simulink model "main"  (R2016b)
settings: Solver=VariableStepAuto  StartTime=0.0  StopTime=0.4  FixedStep=2e-4  RelTol=1e-3
values from neighbouring files (symbols this model uses):
  TsN = 1e-5    (= 1e-05)    [initiateSimulation.m]
undefined symbols (not defined in the file or in its folder): denGc, denGp, numGc, numGp
libraries: simulink x1, model_controller x1
settings Model: Creator=Dai Luyao  LastModifiedBy=Dai Luyao

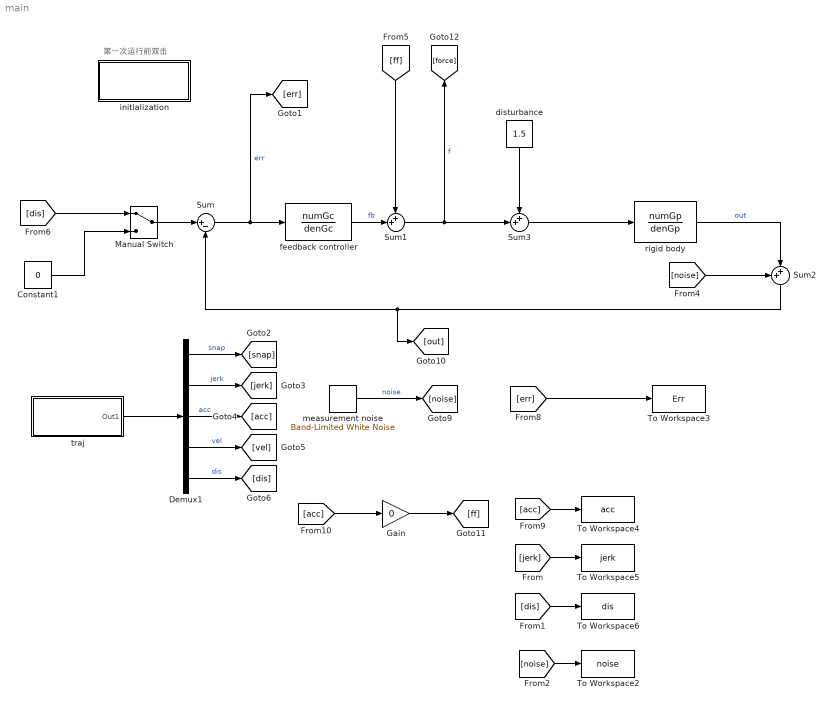
== system main ==
  note: 第一次运行前双击
  Constant1 : Constant  Value=0
  Demux1 : Demux  Outputs=5
  Gain : Gain  Gain=0
  Manual Switch : ManualSwitch
  Sum : Sum  Inputs=|+-
  Sum1 : Sum  Inputs=++|
  Sum2 : Sum  Inputs=++|
  Sum3 : Sum  Inputs=++|
  To Workspace2 : ToWorkspace  VariableName=noise  SaveFormat=Structure With Time  SampleTime=-1
  To Workspace3 : ToWorkspace  VariableName=Err  SaveFormat=Structure With Time  SampleTime=-1
  To Workspace4 : ToWorkspace  VariableName=acc  SaveFormat=Structure With Time  SampleTime=-1
  To Workspace5 : ToWorkspace  VariableName=jerk  SaveFormat=Structure With Time  SampleTime=-1
  To Workspace6 : ToWorkspace  VariableName=dis  SaveFormat=Structure With Time  SampleTime=-1
  disturbance : Constant  Value=1.5
  feedback controller : TransferFcn  Numerator=numGc  Denominator=denGc
  initialization : Subsystem
      settings: OpenFcn=initiateSimulation;  MoveFcn=edit initiateSimulation;
  measurement noise : simulink/Sources/Band-Limited White Noise  Cov=noisePower  Ts=TsN  seed=[23341]
  rigid body : TransferFcn  Numerator=numGp  Denominator=denGp
  traj : Subsystem  BlockChoice=zero
      link override 3rd order traj: j=800  v=0.25  x=0.06  a=10
      link override 4th order traj: a=10  v=0.25
      settings: AttributesFormatString=%<BlockChoice>  TemplateBlock=model_controller/Profile Generators/traj  MemberBlocks=2nd order traj,3rd order traj,4th order traj,step,zero
  wires:
  Sum/1 -> feedback controller/1, [err]  "err"
  feedback controller/1 -> Sum1/2  "fb"
  Sum1/1 -> Sum3/2, [force]  "f"
  measurement noise/1 -> [noise]  "noise"
  rigid body/1 -> Sum2/2  "out"
  Sum2/1 -> [out], Sum/2
  Demux1/1 -> [snap]  "snap"
  Demux1/2 -> [jerk]  "jerk"
  Demux1/3 -> [acc]  "acc"
  Demux1/4 -> [vel]  "vel"
  Demux1/5 -> [dis]  "dis"
  [acc] -> To Workspace4/1
  Gain/1 -> [ff]
  [acc] -> Gain/1
  [jerk] -> To Workspace5/1
  traj/1(Out1) -> Demux1/1
  [ff] -> Sum1/1
  [dis] -> To Workspace6/1
  [err] -> To Workspace3/1
  [noise] -> To Workspace2/1
  Sum3/1 -> rigid body/1
  Manual Switch/1 -> Sum/1
  [dis] -> Manual Switch/1
  [noise] -> Sum2/1
  disturbance/1 -> Sum3/1
  Constant1/1 -> Manual Switch/2

== system main/initialization ==

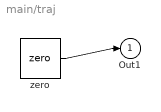
== system main/traj ==
  zero : model_controller/Profile Generators/zero  t=0  v0=0  vf=1  Ts=0
  Out1 : Outport
  wires:
  zero/1 -> Out1/1
